simulink model "commqpskrx"  (R2013b)
settings: Solver=FixedStepDiscrete  SolverMode=SingleTasking  StartTime=0.0  StopTime=1-1e-05  RelTol=1e-3
PreLoadFcn:
  | qpsktxrx = commqpsktxrx_init1();
InitFcn:
  | FrameTime = qpsktxrx.Ts*qpsktxrx.FrameSize*qpsktxrx.Upsampling;
StopFcn:
  | if (strcmp(get_param('commqpskrx/Model Parameters','ShowRecvMsg'),'on'))
  |   if exist('received','var')
  |      commqpsktxrx_bits2char;
  |   else
  |      sprintf('%s\n%s\n%s\n%s','Please run the following two lines of code to get the message output:',...
  |       '>> received = <simOut>.get(''received'');',...
  |       '>> commqpsktxrx_bits2char;',...
  |       'where <simOut> is the output of the sim command.')
  |   end
  | end
undefined symbols (not defined in the file or in its folder): dfilt
libraries: simulink x4, dspsigops x4, commdigbbndpm3 x3, dspstat3 x3, dsparch4 x3, commrflib2 x2, commblksprivate x2, commsequence2 x2, commutil2 x2, commfilt2 x2, dspsrcs4 x2, commchan3 x1
(part 1 of 2)
CloseFcn:
  | clear interp_filter;
  | clear TED;
  | clear NCO_ctrl;
  | clear sdrqpsktxrx;
  | clear received;
  | clear qpsktxrx;
  | clear FrameTime;
Description:
  | QPSK Transmitter and Receiver.
  | 
  | This model shows the implementation of a QPSK transmitter and receiver.
settings Model: FPTRunName=Active  Creator=The MathWorks Inc.  LastModifiedBy=DPu1
settings DataIOCC: SignalLoggingSaveFormat=ModelDataLogs  SaveOutput=off  SaveTime=off
settings OptimizationCC: BooleanDataType=off  InlineParams=on  ExpressionDepthLimit=2147483647  LocalBlockOutputs=off
settings DebuggingCC: AlgebraicLoopMsg=error  MultiTaskDSMMsg=warning  MultiTaskCondExecSysMsg=none  SingleTaskRateTransMsg=error  ParameterPrecisionLossMsg=none  FcnCallInpInsideContextMsg=UseLocalSettings  StateNameClashWarn=warning
settings HardwareCC: TargetLongLongMode=on  TargetIntDivRoundTo=Zero  TargetEndianess=LittleEndian  TargetHWDeviceType=Generic->MATLAB Host Computer  ProdEqTarget=off
settings RTWCC: ProcessScript=grt_make_rtw_hook  IncludeERTFirstTime=on
settings GRTTargetCC: CodeReplacementLibrary=None  CombineOutputUpdateFcns=off  CPPClassGenCompliant=on

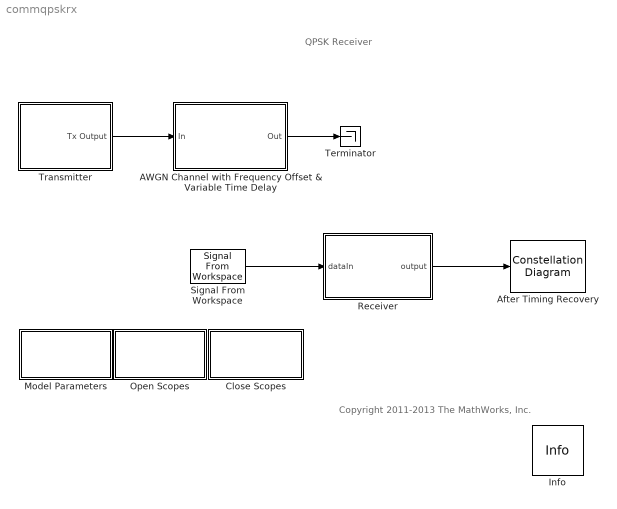
== system commqpskrx ==
  note: QPSK Receiver
  note: Copyright 2011-2013 The MathWorks, Inc.
  AWGN Channel with Frequency Offset & Variable Time Delay : Subsystem
      mask Display: disp('AWGN Channel with\nFrequency Offset & \nVariable Time Delay');
  After Timing Recovery : ConstellationDiagram  Tag=ScatterPlot
      settings: CopyFcn=scopeextensions.ScopeBlock.onCoreBlockCopy(gcbh);  DeleteFcn=scopeextensions.ScopeBlock.callback(gcbh, 'onBlockDelete');  PreSaveFcn=scopeextensions.ScopeBlock.callback(gcbh, 'onModelSave');  NameChangeFcn=scopeextensions.ScopeBlock.callback(gcbh, 'onBlockRename');  DestroyFcn=scopeextensions.ScopeBlock.onBlockDestroy(gcbh)  CloseFcn=scopeextensions.ScopeBlock.callback(gcbh, 'onBlockClose');  PreDeleteFcn=scopeextensions.ScopeBlock.callback(gcbh, 'onBlockPreDelete');
  Close Scopes : Subsystem
      settings: OpenFcn=|
      | % Close the Spectrum Scopes, Time Scopes, and the Scatter Plot Scopes
      | sdspfscope2([],[],[],'ScopeUpdate',[bdroot '/Transmitter/After RC Tx Filter'],'CloseFig');
      | set_param([bdroot '/Transmitter/After RC Tx Filter'],'OpenScopeAtSimStart','off');
      | 
      | channelSubsys = [bdroot '/AWGN Channel with Frequency Offset & Variable Time Delay'];
      | sdspfscope2([],[],[],'ScopeUpdate',[channelSubsys '/After Channel'],'CloseFig');
      | set_param([channelSubsys '/After Channel'],'OpenScopeAtSimStart','off');
      | 
      | TMW_Delay_TimeScope = scopeextensions.ScopeBlock.getInstance([channelSubsys '/Actual Delay']);
      | TMW_Delay_TimeScope.Visible = 'off';
      | TMW_Delay_TimeScope.ScopeCfg.OpenAtMdlStart = false;
      | 
      | sdspfscope2([],[],[],'ScopeUpdate',[bdroot '/Receiver/After RC Rx Filter'],'CloseFig');
      | set_param([bdroot '/Receiver/After RC Rx Filter'],'OpenScopeAtSimStart','off');
      | 
      | sdspfscope2([],[],[],'ScopeUpdate',[bdroot '/Receiver/After RC Rx Filter1'],'CloseFig');
      | set_param([bdroot '/Receiver/After RC Rx Filter1'],'OpenScopeAtSimStart','off');
      | 
      | CoarseFreqCompSubsys = [bdroot '/Receiver/Coarse Frequency Compensation'];
      | TMW_Freq_Offset_TimeScope = scopeextensions.ScopeBlock.getInstance([CoarseFreqCompSubsys '/Estimated Frequency Offset']);
      | TMW_Freq_Offset_TimeScope.Visible = 'off';
      | TMW_Freq_Offset_TimeScope.ScopeCfg.OpenAtMdlStart = false;
      | sdspfscope2([],[],[],'ScopeUpdate',[CoarseFreqCompSubsys '/Find Frequency Offset/After u^M'],'CloseFig');
      | set_param([CoarseFreqCompSubsys '/Find Frequency Offset/After u^M'],'OpenScopeAtSimStart','off');
      | % sdspfscope2([],[],[],'ScopeUpdate',[bdroot '/Receiver/After Coarse Frequency Compensation'],'CloseFig');
      | % set_param([bdroot '/Receiver/After Coarse Frequency Compensation'],'OpenScopeAtSimStart','off');
      | 
      | 
      | FineFreqCompSubsys = [bdroot '/Receiver/Fine Frequency Compensation'];
      | sdspfscope2([],[],[],'ScopeUpdate',[FineFreqCompSubsys '/Estimated Phase Difference'],'CloseFig');
      | set_param([FineFreqCompSubsys '/Estimated Phase Difference'],'OpenScopeAtSimStart','off');
      | 
      | sdspfscope2([],[],[],'ScopeUpdate',[bdroot '/Receiver/After Fine Frequency Compensation'],'CloseFig');
      | set_param([bdroot '/Receiver/After Fine Frequency Compensation'],'OpenScopeAtSimStart','off');
      | 
      | TimeRecSubsys = [bdroot '/Receiver/Timing Recovery'];
      | TMW_Delay_Offset_TimeScope = scopeextensions.ScopeBlock.getInstance([TimeRecSubsys '/Timing Recovery PLL/Normalized Timing Error']);
      | TMW_Delay_Offset_TimeScope.Visible = 'off';
      | TMW_Delay_Offset_TimeScope.ScopeCfg.OpenAtMdlStart = false;
      | 
      | sdspfscope2([],[],[],'ScopeUpdate',[TimeRecSubsys '/After Timing Recovery'],'CloseFig');
      | set_param([TimeRecSubsys '/After Timing Recovery'],'OpenScopeAtSimStart','off');
      | 
      | clear TMW_Delay_TimeScope TMW_Freq_Offset_TimeScope TMW_Delay_Offset_TimeScope;
      | clear channelSubsys CoarseFreqCompSubsys  FineFreqCompSubsys TimeRecSubsys;
      mask Display: disp('Double-click\nTo Close Scopes');
  Info : commblksprivate/Info  SystemSampleTime=-1
  Model Parameters : Subsystem  mask(Model Parameters){SettingCtrl=Timing recovery settings, EbN0dB=7, FreqOffset=5e3, DelayCtrl=Triangle, DelayStep=0.05, MinDelay=0, MaxDelay=8, DelayStart=0.1, FFTSize=2048, numSpecAverage=2, FineFreqNormalizedLoopBW=0.01, FineFreqDampingFactor=1, TimeRecNormalizedLoopBW=0.01, TimeRecDampingFactor=1, ShowRecvMsg=on}
      mask prompts: SettingCtrl "Setting types:"; EbN0dB "Eb/No (dB):"; FreqOffset "Frequency offset (Hz):"; DelayCtrl "Delay type:"; DelayStep "Delay step (samples/frame):"; MinDelay "Minimum delay (samples):"; MaxDelay "Maximum delay (samples):"; DelayStart "Start delay (samples):"; FFTSize "FFT size for coarse frequency compensation:"; numSpecAverage "Number of spectrum averages (frames):"; FineFreqNormalizedLoopBW "Normalized loop bandwidth:"; FineFreqDampingFactor "Damping factor:"; TimeRecNormalizedLoopBW "Normalized loop bandwidth:"; TimeRecDampingFactor "Damping factor:"; ShowRecvMsg "Show received message:"
      mask help: Choose to set the channel impairment parameters, FFT parameters for the coarse frequency compensation, PLL parameters for fine frequency compensation and timing recovery.
      mask init:
      | myException = commqpsktxrx_mask(gcb, 'init', DelayCtrl, MinDelay,...
      |     MaxDelay, DelayStart, DelayStep);
      | if ~isempty(myException)
      |    errordlg(myException.msg);
      | end
      mask Help: helpview(commdhelp);
      mask TypeOptions SettingCtrl: Channel impairment settings | FFT settings for coarse frequency compensation | Fine frequency compensation settings | Timing recovery settings
      mask Callback SettingCtrl: commqpsktxrx_mask(gcbh, 'cbShowHideSettingOptions');
      mask TypeOptions DelayCtrl: Ramp | Triangle
      mask Callback DelayCtrl: commqpsktxrx_mask(gcbh, 'cbShowHideDelayOptions');
      mask Display: disp('Model\nParameters');
  Open Scopes : Subsystem
      settings: OpenFcn=|
      | % Open the Spectrum Scopes, Time Scopes, and the Scatter Plot Scopes
      | sdspfscope2([],[],[],'ScopeUpdate',[bdroot '/Transmitter/After RC Tx Filter'],'OpenFig');
      | set_param([bdroot '/Transmitter/After RC Tx Filter'],'OpenScopeAtSimStart','on');
      | 
      | sdspfscope2([],[],[],'ScopeUpdate',[bdroot '/AWGN Channel with Frequency Offset & Variable Time Delay/After Channel'],'OpenFig');
      | set_param([bdroot '/AWGN Channel with Frequency Offset & Variable Time Delay/After Channel'],'OpenScopeAtSimStart','on');
      | 
      | channelSubsys = [bdroot '/AWGN Channel with Frequency Offset & Variable Time Delay'];
      | TMW_Delay_TimeScope = scopeextensions.ScopeBlock.getInstance([channelSubsys '/Actual Delay']);
      | TMW_Delay_TimeScope.Visible = 'on';
      | TMW_Delay_TimeScope_hs = TMW_Delay_TimeScope.Framework;
      | % Enable the Plot Navigation
      | TMW_Delay_TimeScope_hs.ExtDriver.ConfigDb.findConfig('Tools', 'Plot Navigation').Enable = true;
      | TMW_Delay_TimeScope.Position = figposition([1.5 6.3 22 24]);
      | TMW_Delay_TimeScope.ScopeCfg.OpenAtMdlStart = true;
      | 
      | sdspfscope2([],[],[],'ScopeUpdate',[bdroot '/Receiver/After RC Rx Filter'],'OpenFig');
      | set_param([bdroot '/Receiver/After RC Rx Filter'],'OpenScopeAtSimStart','on');
      | 
      | sdspfscope2([],[],[],'ScopeUpdate',[bdroot '/Receiver/After RC Rx Filter1'],'OpenFig');
      | set_param([bdroot '/Receiver/After RC Rx Filter1'],'OpenScopeAtSimStart','on');
      | 
      | CoarseFreqCompSubsys = [bdroot '/Receiver/Coarse Frequency Compensation'];
      | TMW_Freq_Offset_TimeScope = scopeextensions.ScopeBlock.getInstance([CoarseFreqCompSubsys '/Estimated Frequency Offset']);
      | TMW_Freq_Offset_TimeScope.Visible = 'on';
      | TMW_Freq_Offset_TimeScope_hs = TMW_Freq_Offset_TimeScope.Framework;
      | % Enable the Plot Navigation
      | TMW_Freq_Offset_TimeScope_hs.ExtDriver.ConfigDb.findConfig('Tools', 'Plot Navigation').Enable = true;
      | TMW_Freq_Offset_TimeScope.Position = figposition([24 6.3 22 24]);
      | TMW_Freq_Offset_TimeScope.ScopeCfg.OpenAtMdlStart = true;
      | sdspfscope2([],[],[],'ScopeUpdate',[CoarseFreqCompSubsys '/Find Frequency Offset/After u^M'],'OpenFig');
      | set_param([CoarseFreqCompSubsys '/Find Frequency Offset/After u^M'],'OpenScopeAtSimStart','on');
      | % sdspfscope2([],[],[],'ScopeUpdate',[bdroot '/Receiver/After Coarse Frequency Compensation'],'OpenFig');
      | % set_param([bdroot '/Receiver/After Coarse Frequency Compensation'],'OpenScopeAtSimStart','on');
      | 
      | 
      | FineFreqCompSubsys = [bdroot '/Receiver/Fine Frequency Compensation'];
      | sdspfscope2([],[],[],'ScopeUpdate',[FineFreqCompSubsys '/Estimated Phase Difference'],'OpenFig');
      | set_param([FineFreqCompSubsys '/Estimated Phase Difference'],'OpenScopeAtSimStart','on');
      | 
      | sdspfscope2([],[],[],'ScopeUpdate',[bdroot '/Receiver/After Fine Frequency Compensation'],'OpenFig');
      | set_param([bdroot '/Receiver/After Fine Frequency Compensation'],'OpenScopeAtSimStart','on');
      | 
      | TimeRecSubsys = [bdroot '/Receiver/Timing Recovery'];
      | TMW_Delay_Offset_TimeScope = scopeextensions.ScopeBlock.getInstance([TimeRecSubsys '/Timing Recovery PLL/Normalized Timing Error']);
      | TMW_Delay_Offset_TimeScope.Visible = 'on';
      | TMW_Delay_Offset_TimeScope_hs = TMW_Delay_Offset_TimeScope.Framework;
      | % Enable the Plot Navigation
      | TMW_Delay_Offset_TimeScope_hs.ExtDriver.ConfigDb.findConfig('Tools', 'Plot Navigation').Enable = true;
      | TMW_Delay_Offset_TimeScope.Position = figposition([46.5 6.3 22 24]);
      | TMW_Delay_Offset_TimeScope.ScopeCfg.OpenAtMdlStart = true;
      | 
      | sdspfscope2([],[],[],'ScopeUpdate',[TimeRecSubsys '/After Timing Recovery'],'OpenFig');
      | set_param([TimeRecSubsys '/After Timing Recovery'],'OpenScopeAtSimStart','on');
      | clear TMW_Delay_TimeScope TMW_Freq_Offset_TimeScope TMW_Delay_Offset_TimeScope TMW_Delay_TimeScope_hs TMW_Freq_Offset_TimeScope_hs TMW_Delay_Offset_TimeScope_hs;
      | clear channelSubsys CoarseFreqCompSubsys  FineFreqCompSubsys TimeRecSubsys;
      mask Display: disp('Double-click\nTo Open Scopes\nAt Run Time');
  Receiver : Subsystem
      mask Display: disp('Receiver')
  Signal From Workspace : dspsrcs4/Signal From Workspace  X=rxsignal  Ts=0.002/400  nsamps=400  OutputAfterFinalValue=Cyclic repetition  ignoreOrWarnInputAndFrameLengths=off
  Terminator : Terminator
  Transmitter : Subsystem
      mask Display: disp('Transmitter')
  wires:
  Transmitter/1(Tx Output) -> AWGN Channel with Frequency Offset & Variable Time Delay/1(In)
  AWGN Channel with Frequency Offset & Variable Time Delay/1(Out) -> Terminator/1
  Signal From Workspace/1 -> Receiver/1(dataIn)
  Receiver/1(output) -> After Timing Recovery/1

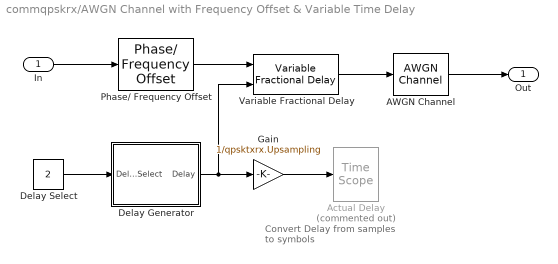
== system commqpskrx/AWGN Channel with Frequency Offset & Variable Time Delay ==
  note: Convert Delay from
      | samples to symbols
  In : Inport
  AWGN Channel : commchan3/AWGN Channel  InputProcessing=Inherited (this choice will be removed - see release notes)  seed=67  noiseMode="Signal to noise ratio  (Eb/No)"  EbNodB=7  EsNodB=15  SNRdB=15  bitsPerSym=2  Ps=1/qpsktxrx.Upsampling  Tsym=qpsktxrx.Upsampling*qpsktxrx.Ts  variance=1
  Actual Delay : TimeScope  Commented=on  DefaultConfigurationName=spbscopes.TimeScopeBlockCfg
      settings: CopyFcn=scopeextensions.ScopeBlock.onCoreBlockCopy(gcbh);  DeleteFcn=scopeextensions.ScopeBlock.callback(gcbh, 'onBlockDelete');  PreSaveFcn=scopeextensions.ScopeBlock.callback(gcbh, 'onModelSave');  NameChangeFcn=scopeextensions.ScopeBlock.callback(gcbh, 'onBlockRename');  DestroyFcn=scopeextensions.ScopeBlock.onBlockDestroy(gcbh)  CloseFcn=scopeextensions.ScopeBlock.callback(gcbh, 'onBlockClose');  PreDeleteFcn=scopeextensions.ScopeBlock.callback(gcbh, 'onBlockPreDelete');
  Delay Generator : Subsystem
      mask Display: disp('Delay Generator')
  Delay Select : Constant  Value=2
  Gain : Gain  Gain=1/qpsktxrx.Upsampling
  Phase/ Frequency Offset : commrflib2/Phase// Frequency Offset  phaseOffset=qpsktxrx.PhaseOffset  freqPort=off  freqOffset=5000
  Variable Fractional Delay : dspsigops/Variable Fractional Delay  mode=OBSOLETE  modeActive=Linear  dmax=qpsktxrx.FrameSize*qpsktxrx.Upsampling  InputProcessing=Columns as channels (frame based)  L=4  FarrowL=4  R=10  alpha=1  ic=0  fallbackFIR=Clip to the minimum value necessary for centered kernel  fallbackFarrow=Clip to the minimum value necessary for centered kernel  noDFT=off  roundingMode=Zero  overflowMode=off
  Out : Outport
  wires:
  AWGN Channel/1 -> Out/1
  In/1 -> Phase/ Frequency Offset/1
  Phase/ Frequency Offset/1 -> Variable Fractional Delay/1
  Variable Fractional Delay/1 -> AWGN Channel/1
  Delay Select/1 -> Delay Generator/1(Delay Select)
  Delay Generator/1(Delay) -> Variable Fractional Delay/2, Gain/1
  Gain/1 -> Actual Delay/1

== system commqpskrx/Close Scopes ==

== system commqpskrx/Model Parameters ==

== system commqpskrx/Open Scopes ==

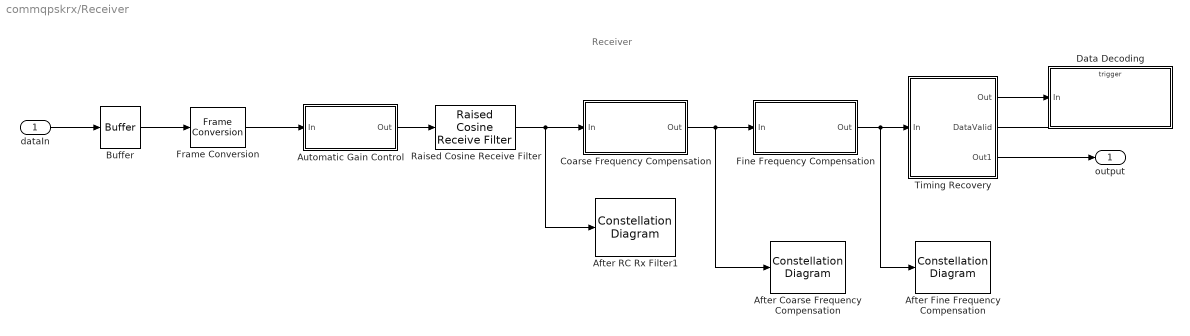
== system commqpskrx/Receiver ==
  note: Receiver
  dataIn : Inport
  After Coarse Frequency Compensation : ConstellationDiagram  Tag=ScatterPlot
      settings: CopyFcn=scopeextensions.ScopeBlock.onCoreBlockCopy(gcbh);  DeleteFcn=scopeextensions.ScopeBlock.callback(gcbh, 'onBlockDelete');  PreSaveFcn=scopeextensions.ScopeBlock.callback(gcbh, 'onModelSave');  NameChangeFcn=scopeextensions.ScopeBlock.callback(gcbh, 'onBlockRename');  DestroyFcn=scopeextensions.ScopeBlock.onBlockDestroy(gcbh)  CloseFcn=scopeextensions.ScopeBlock.callback(gcbh, 'onBlockClose');  PreDeleteFcn=scopeextensions.ScopeBlock.callback(gcbh, 'onBlockPreDelete');
  After Fine Frequency Compensation : ConstellationDiagram  Tag=ScatterPlot
      settings: CopyFcn=scopeextensions.ScopeBlock.onCoreBlockCopy(gcbh);  DeleteFcn=scopeextensions.ScopeBlock.callback(gcbh, 'onBlockDelete');  PreSaveFcn=scopeextensions.ScopeBlock.callback(gcbh, 'onModelSave');  NameChangeFcn=scopeextensions.ScopeBlock.callback(gcbh, 'onBlockRename');  DestroyFcn=scopeextensions.ScopeBlock.onBlockDestroy(gcbh)  CloseFcn=scopeextensions.ScopeBlock.callback(gcbh, 'onBlockClose');  PreDeleteFcn=scopeextensions.ScopeBlock.callback(gcbh, 'onBlockPreDelete');
  After RC Rx Filter1 : ConstellationDiagram  Tag=ScatterPlot
      settings: CopyFcn=scopeextensions.ScopeBlock.onCoreBlockCopy(gcbh);  DeleteFcn=scopeextensions.ScopeBlock.callback(gcbh, 'onBlockDelete');  PreSaveFcn=scopeextensions.ScopeBlock.callback(gcbh, 'onModelSave');  NameChangeFcn=scopeextensions.ScopeBlock.callback(gcbh, 'onBlockRename');  DestroyFcn=scopeextensions.ScopeBlock.onBlockDestroy(gcbh)  CloseFcn=scopeextensions.ScopeBlock.callback(gcbh, 'onBlockClose');  PreDeleteFcn=scopeextensions.ScopeBlock.callback(gcbh, 'onBlockPreDelete');
  Automatic Gain Control : Subsystem  mask{DesiredAmplitude=1/sqrt(qpsktxrx.Upsampling)}
      mask prompts: DesiredAmplitude "Desired Amplitude"
      mask Display: disp('Automatic Gain\nControl')
  Buffer : Buffer  N=qpsktxrx.RxBufferedFrames*qpsktxrx.FrameSize*qpsktxrx.Upsampling  TreatMby1Signals=One channel
  Coarse Frequency Compensation : Subsystem
      mask Display: disp('Coarse Frequency\nCompensation');
  Data Decoding : Subsystem
      mask Display: disp('Data Decoding');
  Fine Frequency Compensation : Subsystem
      mask Display: disp('Fine Frequency\nCompensation')
  Frame Conversion : FrameConversion  OutFrame=Sample-based
  Raised Cosine Receive Filter : commfilt2/Raised Cosine Receive Filter  filtType=Square root  N=qpsktxrx.Upsampling  filtSpan=qpsktxrx.RaisedCosineFilterSpan  currentFiltSpan=qpsktxrx.RaisedCosineFilterSpan  D=(qpsktxrx.RaisedCosineFilterSpan)/2  R=0.5  sampMode=Mute  saveAsFlag=0  rateMode=Downsampling  downFactor=qpsktxrx.Downsampling  downOffset=0  framing=Enforce single-rate processing  InputProcessing=Columns as channels (frame based)  checkGain=Normalized  filterGain=1  checkCoeff=off  variableName=rcRxFilt1  launchFVT=off  roundingMode=Floor  overflowMode=off
  Timing Recovery : Subsystem
      mask Display:
      | disp('Timing\nRecovery');
      | port_label('output',1,'DataOut');
      | port_label('output',2,'DataValid');
  output : Outport
  wires:
  Timing Recovery/1(Out) -> Data Decoding/1(In)
  dataIn/1 -> Buffer/1
  Timing Recovery/2(DataValid) -> Data Decoding/Trigger
  Raised Cosine Receive Filter/1 -> Coarse Frequency Compensation/1(In), After RC Rx Filter1/1
  Coarse Frequency Compensation/1(Out) -> Fine Frequency Compensation/1(In), After Coarse Frequency Compensation/1
  Fine Frequency Compensation/1(Out) -> Timing Recovery/1(In), After Fine Frequency Compensation/1
  Buffer/1 -> Frame Conversion/1
  Frame Conversion/1 -> Automatic Gain Control/1(In)
  Automatic Gain Control/1(Out) -> Raised Cosine Receive Filter/1
  Timing Recovery/3(Out1) -> output/1

== system commqpskrx/Transmitter ==
  note: Transmitter
  Bit Generation : Subsystem
      mask Display: disp('Bits Generation')
  QPSK Modulator Baseband : commdigbbndpm3/QPSK Modulator Baseband  InType=Bit  Enc=Gray  Ph=pi/4  outDtype=double  outWordLen=16  outUDDataType=sfix(16)  outFracLenMode=Best precision  outFracLen=15
  Raised Cosine Transmit Filter : commfilt2/Raised Cosine Transmit Filter  filtType=Square root  filtSpan=qpsktxrx.RaisedCosineFilterSpan  currentFiltSpan=qpsktxrx.RaisedCosineFilterSpan  D=(qpsktxrx.RaisedCosineFilterSpan)/2  R=0.5  sampMode=Mute  saveAsFlag=0  N=qpsktxrx.Upsampling  framing=Enforce single-rate processing  InputProcessing=Columns as channels (frame based)  checkGain=Normalized  filterGain=1  checkCoeff=off  variableName=rcTxFilt  launchFVT=off  roundingMode=Floor  overflowMode=off
  Tx Output : Outport
  wires:
  Bit Generation/1(Out) -> QPSK Modulator Baseband/1
  QPSK Modulator Baseband/1 -> Raised Cosine Transmit Filter/1
  Raised Cosine Transmit Filter/1 -> Tx Output/1

== system commqpskrx/AWGN Channel with Frequency Offset & Variable Time Delay/Delay Generator ==
  Delay Select : Inport
  Multiport Switch : MultiPortSwitch  Inputs=2  OutDataTypeStr=double
  Repeating Sequence Stair : simulink/Sources/Repeating Sequence Stair  OutValues="[0        0.05         0.1        0.15         0.2        0.25         0.3        0.35         0.4        0.45         0.5        0.55         0.6        0.65         0.7        0.75         0.8        0.85         0.9        0.95           1        1.05         1.1        1.15         1.2        1.25         1.3        1.35         1.4        1.45         1.5        1.55         1.6        1.65         1.7        1.75         1.8        1.85         1.9        1.95           2        2.05         2.1        2.15         2.2        2.25         2.3        2.35         2.4        2.45         2.5        2.55         2.6        2.65         2.7        2.75         2.8        2.85         2.9        2.95           3        3.05         3.1        3.15         3.2        3.25         3.3        3.35         3.4        3.45         3.5        3.55         3.6        3.65         3.7        3.75         3.8        3.85         3.9        3.95           4        4.05         4.1        4.15         4.2        4.25         4.3        4.35         4.4        4.45         4.5        4.55         4.6        4.65         4.7        4.75         4.8        4.85         4.9        4.95           5        5.05         5.1        5.15         5.2        5.25         5.3        5.35         5.4        5.45         5.5        5.55         5.6        5.65         5.7        5.75         5.8        5.85         5.9        5.95           6        6.05         6.1        6.15         6.2        6.25         6.3        6.35         6.4        6.45         6.5        6.55         6.6        6.65         6.7        6.75         6.8        6.85         6.9        6.95           7        7.05         7.1        7.15         7.2        7.25         7.3        7.35         7.4        7.45         7.5        7.55         7.6        7.65         7.7        7.75         7.8        7.85         7.9        7.95           8        7.95         7.9        7.85         7.8        7.75         7.7        7.65         7.6        7.55         7.5        7.45         7.4        7.35         7.3        7.25         7.2        7.15         7.1        7.05           7        6.95         6.9        6.85         6.8        6.75         6.7        6.65         6.6        6.55         6.5        6.45         6.4        6.35         6.3        6.25         6.2        6.15         6.1        6.05           6        5.95         5.9        5.85         5.8        5.75         5.7        5.65         5.6        5.55         5.5        5.45         5.4        5.35         5.3        5.25         5.2        5.15         5.1        5.05           5        4.95         4.9        4.85         4.8        4.75         4.7        4.65         4.6        4.55         4.5        4.45         4.4        4.35         4.3        4.25         4.2        4.15         4.1        4.05           4        3.95         3.9        3.85         3.8        3.75         3.7        3.65         3.6        3.55         3.5        3.45         3.4        3.35         3.3        3.25         3.2        3.15         3.1        3.05           3        2.95         2.9        2.85         2.8        2.75         2.7        2.65         2.6        2.55         2.5        2.45         2.4        2.35         2.3        2.25         2.2        2.15         2.1        2.05           2        1.95         1.9        1.85         1.8        1.75         1.7        1.65         1.6        1.55         1.5        1.45         1.4        1.35         1.3        1.25         1.2        1.15         1.1        1.05           1        0.95         0.9        0.85         0.8        0.75         0.7        0.65         0.6        0.55         0.5        0.45         0.4        0.35         0.3        0.25         0.2        0.15         0.1        0.05]"  tsamp=qpsktxrx.FrameSize*qpsktxrx.Upsampling*qpsktxrx.Ts  OutMin=[]  OutMax=[]  OutDataTypeStr=double  OutputDataTypeScalingMode=double  OutDataType=fixdt(0,8)  ConRadixGroup=Best Precision: Vector-wise  OutScaling=2^-12
  mVariableRamp : Subsystem
  Delay : Outport
  wires:
  Delay Select/1 -> Multiport Switch/1
  Repeating Sequence Stair/1 -> Multiport Switch/3
  mVariableRamp/1(Out) -> Multiport Switch/2
  Multiport Switch/1 -> Delay/1

== system commqpskrx/Receiver/Automatic Gain Control ==
  In : Inport
  AGC : commrfcorlib/AGC  SimulateUsing=Interpreted execution  DetectorMethod=Rectifier  LoopMethod=Linear  UpdatePeriod=32  StepSize=0.5  MaximumGain=20  GainOutputPort=off
  Gain : Gain  Gain=DesiredAmplitude
  Out : Outport
  wires:
  In/1 -> AGC/1
  Gain/1 -> Out/1
  AGC/1 -> Gain/1

== system commqpskrx/Receiver/Coarse Frequency Compensation ==
  In : Inport
  Compensate for Frequency Offset : commrflib2/Phase// Frequency Offset  phaseOffset=0  freqPort=on  freqOffset=100
  Estimated Frequency Offset : TimeScope  Commented=on  DefaultConfigurationName=spbscopes.TimeScopeBlockCfg
      settings: CopyFcn=scopeextensions.ScopeBlock.onCoreBlockCopy(gcbh);  DeleteFcn=scopeextensions.ScopeBlock.callback(gcbh, 'onBlockDelete');  PreSaveFcn=scopeextensions.ScopeBlock.callback(gcbh, 'onModelSave');  NameChangeFcn=scopeextensions.ScopeBlock.callback(gcbh, 'onBlockRename');  DestroyFcn=scopeextensions.ScopeBlock.onBlockDestroy(gcbh)  CloseFcn=scopeextensions.ScopeBlock.callback(gcbh, 'onBlockClose');  PreDeleteFcn=scopeextensions.ScopeBlock.callback(gcbh, 'onBlockPreDelete');
  Find Frequency Offset : Subsystem
  Gain : Gain  Gain=-1
  Out : Outport
  wires:
  Find Frequency Offset/1(Freq Offset) -> Gain/1, Estimated Frequency Offset/1
  In/1 -> Compensate for Frequency Offset/1, Find Frequency Offset/1(In)
  Compensate for Frequency Offset/1 -> Out/1
  Gain/1 -> Compensate for Frequency Offset/2

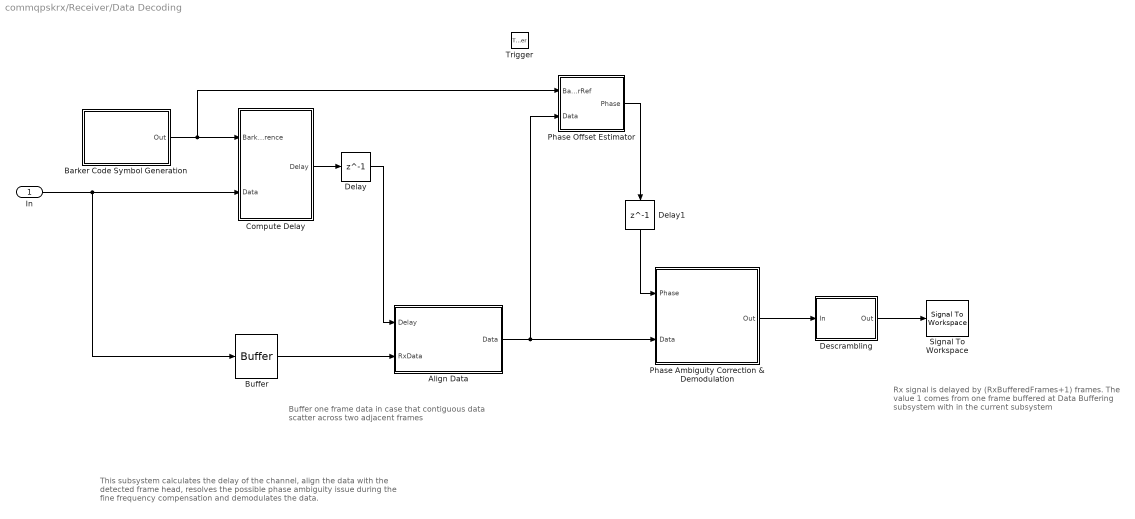
== system commqpskrx/Receiver/Data Decoding ==
  note: Buffer one frame data in case that contiguous
      | data scatter across two adjacent frames
  note: This subsystem calculates the delay of the channel, align the data with
      | the detected frame head, resolves the possible phase ambiguity issue
      | during the fine frequency compensation and demodulates the data.
  note: Rx signal is delayed by (RxBufferedFrames+1) frames.
      | The value 1 comes from one frame buffered at Data
      | Buffering subsystem with in the current subsystem
  In : Inport
  Trigger : TriggerPort  PortDimensions=1
  Align Data : MATLAB Function  TreatAsAtomicUnit=on
  "Barker Code Symbol Generation " : Subsystem
      mask Display: disp('Barker Code\nSymbol Generation')
  Buffer : Buffer  N=qpsktxrx.FrameSize*2  V=qpsktxrx.FrameSize  TreatMby1Signals=One channel
  Compute Delay : Subsystem
      mask Display: disp('Compute\nDelay');
  Delay : Delay  DelayLength=1
  Delay1 : Delay  DelayLength=1
  Descrambling : Subsystem
      mask Display: disp('Descrambling');
  Phase Ambiguity Correction & Demodulation : Subsystem
      mask Display: disp('Phase Ambiguity\nCorrection\n& Demodulation');
  Phase Offset Estimator : Subsystem
  Signal To Workspace : SignalToWorkspace  VariableName=received
      settings: CopyFcn=dspblkcopystw(gcbh);
  wires:
  Delay/1 -> Align Data/1(Delay)
  Buffer/1 -> Align Data/2(RxData)
  In/1 -> Compute Delay/2(Data), Buffer/1
  Compute Delay/1(Delay) -> Delay/1
  Align Data/1(Data) -> Phase Ambiguity Correction & Demodulation/2(Data), Phase Offset Estimator/2(Data)
  Phase Ambiguity Correction & Demodulation/1(Out) -> Descrambling/1(In)
  "Barker Code Symbol Generation "/1(Out) -> Compute Delay/1(Barker Reference), Phase Offset Estimator/1(BarkerRef)
  Phase Offset Estimator/1(Phase) -> Delay1/1
  Delay1/1 -> Phase Ambiguity Correction & Demodulation/1(Phase)
  Descrambling/1(Out) -> Signal To Workspace/1

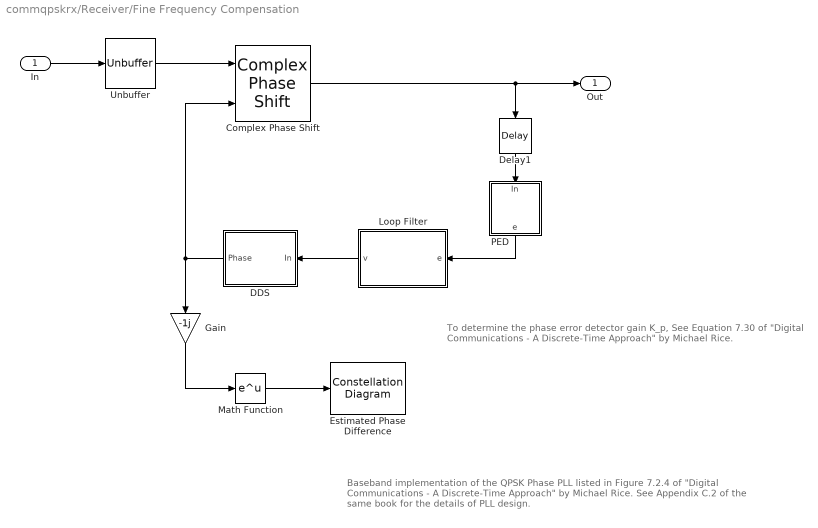
== system commqpskrx/Receiver/Fine Frequency Compensation ==
  note: To determine the phase error detector gain K_p, See Equation 7.30 of "Digital
      | Communications - A Discrete-Time Approach" by Michael Rice.
  note: Baseband implementation of the QPSK Phase PLL listed in Figure 7.2.4 of
      | "Digital Communications - A Discrete-Time Approach" by Michael Rice. See
      | Appendix C.2 of the same book for the details of PLL design.
  In : Inport
  Complex Phase Shift : commutil2/Complex Phase Shift
  DDS : Subsystem
      mask Display: disp('DDS')
  Delay1 : dspsigops/Delay  InputProcessing=Columns as channels (frame based)  dly_unit=Samples  delay=1  ic_detail=off  dif_ic_for_ch=off  dif_ic_for_dly=off  ic=0  reset_popup=None
  Estimated Phase Difference : ConstellationDiagram  Tag=ScatterPlot
      settings: CopyFcn=scopeextensions.ScopeBlock.onCoreBlockCopy(gcbh);  DeleteFcn=scopeextensions.ScopeBlock.callback(gcbh, 'onBlockDelete');  PreSaveFcn=scopeextensions.ScopeBlock.callback(gcbh, 'onModelSave');  NameChangeFcn=scopeextensions.ScopeBlock.callback(gcbh, 'onBlockRename');  DestroyFcn=scopeextensions.ScopeBlock.onBlockDestroy(gcbh)  CloseFcn=scopeextensions.ScopeBlock.callback(gcbh, 'onBlockClose');  PreDeleteFcn=scopeextensions.ScopeBlock.callback(gcbh, 'onBlockPreDelete');
  Gain : Gain  Gain=-1j
  Loop Filter : Subsystem  mask{BnTs=0.01, zeta=1, N=qpsktxrx.Upsampling/qpsktxrx.Downsampling, Kp=qpsktxrx.PhaseErrorDetectorGain, K0=qpsktxrx.PhaseRecoveryGain}
      mask prompts: BnTs "Normalized Loop Bandwidth"; zeta "Damping Factor"; N "Number of Samples/Symbol"; Kp "Phase Detector Gain (Kp)"; K0 "DDS Gain (K0)"
      mask init:
      | % See C.57 to C.61 in Michael Rice's "Digital Communications 
      | % - A Discrete-Time Approach" for details
      | theta = BnTs/(zeta+0.25/zeta)/N;
      | d = 1 + 2*zeta*theta + theta*theta;
      | K1 = 4*zeta*theta/d;
      | K2 = 4*theta*theta/d;
      | K1 = K1/(Kp*K0);
      | K2 = K2/(Kp*K0);
      mask Display: disp('Loop Filter')
  Math Function : Math  SaturateOnIntegerOverflow=on
  PED : MATLAB Function  TreatAsAtomicUnit=on
  Unbuffer : Unbuffer  SampleBasedProcessing=Same as frame based
  Out : Outport
  wires:
  Gain/1 -> Math Function/1
  Math Function/1 -> Estimated Phase Difference/1
  PED/1(e) -> Loop Filter/1(e)
  Loop Filter/1(v) -> DDS/1(In)
  DDS/1(Phase) -> Complex Phase Shift/2, Gain/1
  In/1 -> Unbuffer/1
  Complex Phase Shift/1 -> Delay1/1, Out/1
  Delay1/1 -> PED/1(In)
  Unbuffer/1 -> Complex Phase Shift/1

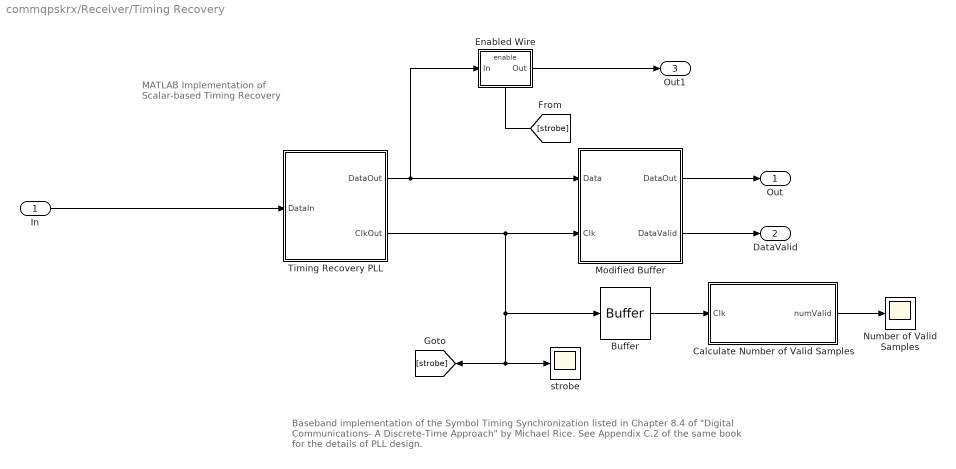
== system commqpskrx/Receiver/Timing Recovery ==
  note: Baseband implementation of the Symbol Timing Synchronization listed in Chapter 8.4
      | of "Digital Communications- A Discrete-Time Approach" by Michael Rice. See
      | Appendix C.2 of the same book for the details of PLL design.
  note: MATLAB Implementation
      | of Scalar-based Timing Recovery
  In : Inport
  Buffer : Buffer  N=qpsktxrx.FrameSize*qpsktxrx.Upsampling/qpsktxrx.Downsampling  TreatMby1Signals=One channel
  Calculate Number of Valid Samples : MATLAB Function  TreatAsAtomicUnit=on
  Enabled Wire : Subsystem  TreatAsAtomicUnit=on
  Modified Buffer : Subsystem  TreatAsAtomicUnit=on  mask(Input-Driven Buffer){bufSize=qpsktxrx.FrameSize}
      mask prompts: bufSize "Buffer size:"
      mask help: A modified buffer subsystem that is driven by the arrival of its input data; it produces a valid output data buffer whenever its buffer is full and sets its dataValid flag to 1. Otherwise, the data at its dataOut port is not valid and its dataValid flag is set to 0.
      mask Display: disp('Modified Buffer')
  Number of Valid Samples : Scope
      settings: TimeRange=0.1  YMin=95  YMax=105  SaveName=ScopeData3  MaxDataPoints=50000
  Timing Recovery PLL : Subsystem
      mask Display:
      | disp('Timing Recovery\nPLL')
      | port_label('input',1,'In')
      | port_label('output',1,'DataOut')
      | port_label('output',2,'Clk')
  strobe : Scope
  Out : Outport
  DataValid : Outport  Port=2
  Out1 : Outport  Port=3
  wires:
  Timing Recovery PLL/2(ClkOut) -> [strobe], strobe/1, Buffer/1, Modified Buffer/2(Clk)
  Timing Recovery PLL/1(DataOut) -> Enabled Wire/1(In), Modified Buffer/1(Data)
  Calculate Number of Valid Samples/1(numValid) -> Number of Valid Samples/1
  [strobe] -> Enabled Wire/Enable
  In/1 -> Timing Recovery PLL/1(DataIn)
  Modified Buffer/1(DataOut) -> Out/1
  Modified Buffer/2(DataValid) -> DataValid/1
  Buffer/1 -> Calculate Number of Valid Samples/1(Clk)
  Enabled Wire/1(Out) -> Out1/1

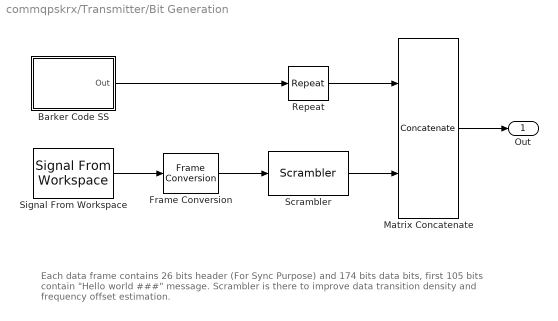
== system commqpskrx/Transmitter/Bit Generation ==
  note: Each data frame contains 26 bits header (For Sync Purpose) and 174 bits data bits,
      | first 105 bits contain "Hello world ###" message. Scrambler is there to improve data
      | transition density and frequency offset estimation.
  Barker Code SS : Subsystem
      mask Display: disp('Unipolar\nBarker Code')
  Frame Conversion : FrameConversion  OutFrame=Sample-based
  Matrix Concatenate : Concatenate  Mode=Multidimensional array
  Repeat : dspsigops/Repeat  N=2  InputProcessing=Columns as channels (frame based)  RateOptions=Enforce single-rate processing  ic=0  mode=Unused parameter value
  Scrambler : commsequence2/Scrambler  M=2  poly=[1 1 1 0 1]  ini_sta=[0 0 0 0]
  Signal From Workspace : dspsrcs4/Signal From Workspace  X=qpsktxrx.sBit  Ts=1/qpsktxrx.DataLength*FrameTime  nsamps=qpsktxrx.DataLength  OutputAfterFinalValue=Cyclic repetition  ignoreOrWarnInputAndFrameLengths=off
  Out : Outport
  wires:
  Barker Code SS/1(Out) -> Repeat/1
  Matrix Concatenate/1 -> Out/1
  Signal From Workspace/1 -> Frame Conversion/1
  Repeat/1 -> Matrix Concatenate/1
  Scrambler/1 -> Matrix Concatenate/2
  Frame Conversion/1 -> Scrambler/1

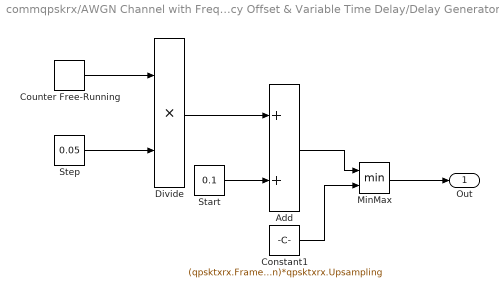
== system commqpskrx/AWGN Channel with Frequency Offset & Variable Time Delay/Delay Generator/mVariableRamp ==
  Add : Sum
  Constant1 : Constant  Value=(qpsktxrx.FrameSize-qpsktxrx.RaisedCosineFilterSpan)*qpsktxrx.Upsampling
  Counter Free-Running : simulink/Sources/Counter Free-Running  NumBits=64  tsamp=qpsktxrx.FrameSize*qpsktxrx.Upsampling*qpsktxrx.Ts
  Divide : Product  Inputs=**
  MinMax : MinMax  Inputs=2
  Start : Constant  Value=0.1
  Step : Constant  Value=0.05
  Out : Outport
  wires:
  Counter Free-Running/1 -> Divide/1
  Step/1 -> Divide/2
  Divide/1 -> Add/1
  Start/1 -> Add/2
  Add/1 -> MinMax/1
  MinMax/1 -> Out/1
  Constant1/1 -> MinMax/2

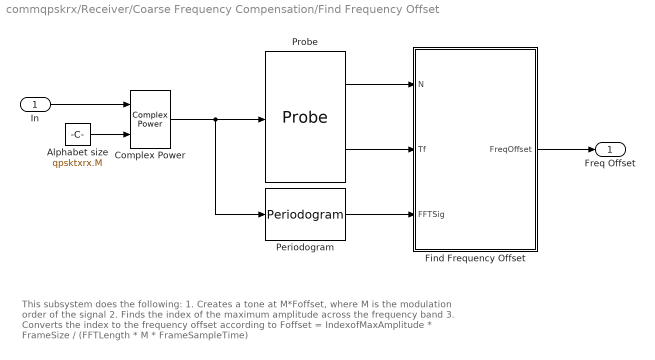
== system commqpskrx/Receiver/Coarse Frequency Compensation/Find Frequency Offset ==
  note: This subsystem does the following:
      | 1.  Creates a tone at M*Foffset, where M is the modulation order of the signal
      | 2.  Finds the index of the maximum amplitude across the frequency band
      | 3.  Converts the index to the frequency offset according to
      | Foffset = IndexofMaxAmplitude * FrameSize / (FFTLength * M * FrameSampleTime)
  In : Inport
  Alphabet size : Constant  Value=qpsktxrx.M  OutDataTypeStr=Inherit: Inherit via back propagation
  Complex Power : commblksprivate/Complex Power
  Find Frequency Offset : MATLAB Function  TreatAsAtomicUnit=on
  Periodogram : dspspect3/Periodogram  measurement=Power spectral density  wintype=Hamming  Rs=50  beta=5  winsamp=Symmetric  FFTImplementation=Auto  inheritFFT=off  fftsize=2048  navg=2  inheritTs=on  Ts=1
  Probe : Probe  ProbeComplexSignal=off
  Freq Offset : Outport
  wires:
  Periodogram/1 -> Find Frequency Offset/3(FFTSig)
  Alphabet size/1 -> Complex Power/2
  In/1 -> Complex Power/1
  Probe/1 -> Find Frequency Offset/1(N)
  Probe/2 -> Find Frequency Offset/2(Tf)
  Find Frequency Offset/1(FreqOffset) -> Freq Offset/1
  Complex Power/1 -> Probe/1, Periodogram/1

== system commqpskrx/Receiver/Data Decoding/Barker Code Symbol Generation  ==
  note: Regenerate a QPSK-modulated unipolar Barker code sequence
      | to be compared with the received data
  Constant Barker Code : Constant  Value=|  VectorParams1D=off  OutDataTypeStr=double
      | [+1 +1 +1 +1 +1 -1 -1 +1 +1 -1 +1 -1 +1
      | ].' > 0
  QPSK Modulator Baseband : commdigbbndpm3/QPSK Modulator Baseband  InType=Bit  Enc=Gray  Ph=pi/4  outDtype=double  outWordLen=16  outUDDataType=sfix(16)  outFracLenMode=Best precision  outFracLen=15
  Repeat : dspsigops/Repeat  N=2  InputProcessing=Columns as channels (frame based)  RateOptions=Enforce single-rate processing  ic=0  mode=Unused parameter value
  Out : Outport
  wires:
  Constant Barker Code/1 -> Repeat/1
  Repeat/1 -> QPSK Modulator Baseband/1
  QPSK Modulator Baseband/1 -> Out/1

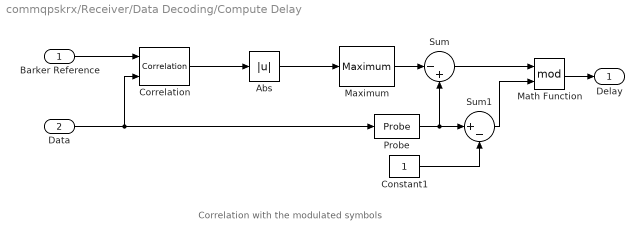
== system commqpskrx/Receiver/Data Decoding/Compute Delay ==
  note: Correlation with the modulated symbols
  Barker Reference : Inport
  Data : Inport  Port=2
  Abs : Abs
  Constant1 : Constant  VectorParams1D=off  OutDataTypeStr=Inherit: Inherit via back propagation  FramePeriod=2
  Correlation : dspstat3/Correlation  domain=Time  outputDataTypeStr=Inherit: Same as accumulator  outputLastDataTypeStr=Inherit: Same as accumulator  outputMin=[]  outputMax=[]  accumDataTypeStr=Inherit: Same as product output  accumLastDataTypeStr=Inherit: Same as product output  roundingMode=Floor  overflowMode=off
  Math Function : Math  Operator=mod  SaturateOnIntegerOverflow=on
  Maximum : dspstat3/Maximum  fcn=Index  reset=None  InputProcessing=Columns as channels (frame based)  indexBase=One  operateOver=Each column  Dimension=1  colComp=on  operation=maximum  roiEnable=off  roiType=Rectangles  roiPortion=Entire ROI  roiOutput=Individual statistics for each ROI  roiFlag=off  accumDataTypeStr=Inherit: Same as product output  accumLastDataTypeStr=Inherit: Same as product output  roundingMode=Floor  overflowMode=off
  Probe : Probe  ProbeSampleTime=off  ProbeComplexSignal=off
  Sum : Sum  Inputs=|-+  SaturateOnIntegerOverflow=on  InputSameDT=on  OutDataTypeStr=Inherit: Same as first input
  Sum1 : Sum  Inputs=|+-  SaturateOnIntegerOverflow=on  InputSameDT=on  OutDataTypeStr=Inherit: Same as first input
  Delay : Outport
  wires:
  Abs/1 -> Maximum/1
  Constant1/1 -> Sum1/2
  Sum1/1 -> Math Function/2
  Math Function/1 -> Delay/1
  Sum/1 -> Math Function/1
  Probe/1 -> Sum1/1, Sum/2
  Correlation/1 -> Abs/1
  Maximum/1 -> Sum/1
  Barker Reference/1 -> Correlation/1
  Data/1 -> Correlation/2, Probe/1

== system commqpskrx/Receiver/Data Decoding/Descrambling ==
  In : Inport
  Descrambler : commsequence2/Descrambler  M=2  poly=[1 1 1 0 1]  ini_sta=[0 0 0 0]
  Selector : Selector  IndexOptions=Index vector (dialog)  Indices=[qpsktxrx.BarkerLength*log2(qpsktxrx.M)+1:qpsktxrx.FrameSize*log2(qpsktxrx.M)]  OutputSizes=1
  Selector1 : Selector  IndexOptions=Index vector (dialog)  Indices=[1:qpsktxrx.MessageLength]  OutputSizes=1
  Out : Outport
  wires:
  Descrambler/1 -> Selector1/1
  Selector1/1 -> Out/1
  In/1 -> Selector/1
  Selector/1 -> Descrambler/1

== system commqpskrx/Receiver/Data Decoding/Phase Ambiguity Correction & Demodulation ==
  note: Phase Ambiguity Resolution
      | and Demodulation
  Phase : Inport
  Data : Inport  Port=2
  Complex Phase Shift : commutil2/Complex Phase Shift
  Gain : Gain  Gain=-1  OutDataTypeStr=Inherit: Same as input
  QPSK Demodulator Baseband : commdigbbndpm3/QPSK Demodulator Baseband  Ph=pi/4  Dec=Gray  OutType=Bit  DecType=Hard decision  VarSource=Dialog  Variance=1  outDtype1=Inherit via internal rule  outDtype2=Inherit via internal rule  derotateFactorWordLen=16
  Out : Outport
  wires:
  Phase/1 -> Gain/1
  Data/1 -> Complex Phase Shift/1
  Complex Phase Shift/1 -> QPSK Demodulator Baseband/1
  QPSK Demodulator Baseband/1 -> Out/1
  Gain/1 -> Complex Phase Shift/2

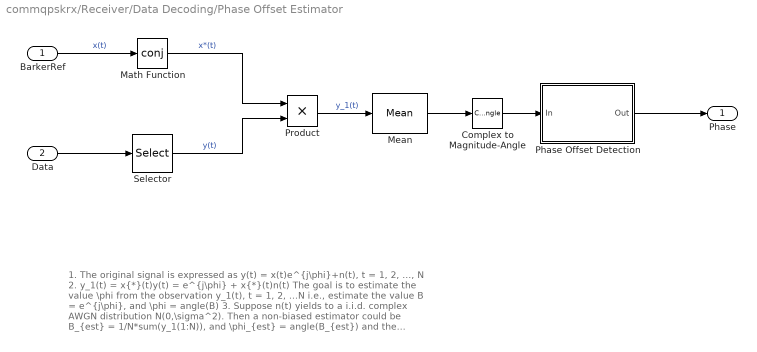
== system commqpskrx/Receiver/Data Decoding/Phase Offset Estimator ==
  note: 1. The original signal is expressed as y(t) = x(t)e^{j\phi}+n(t), t = 1, 2, ..., N
      | 2. y_1(t) = x{*}(t)y(t) = e^{j\phi} + x{*}(t)n(t)
      | The goal is to estimate the value \phi from the observation y_1(t), t = 1, 2, ...N
      | i.e., estimate the value B = e^{j\phi}, and \phi = angle(B)
      | 3. Suppose n(t) yields to a i.i.d. complex AWGN distribution N(0,\sigma^2).
      | Then a non-biased estimator could be
      | B_{est} = 1/N*sum(y_1(1:N)), and \phi_{est} = angle(B_{est})
      | and the variance of B_{est} is \sigma^2/N
  BarkerRef : Inport
  Data : Inport  Port=2
  Complex to Magnitude-Angle : ComplexToMagnitudeAngle  Output=Angle
  Math Function : Math  Operator=conj  SaturateOnIntegerOverflow=on
  Mean : dspstat3/Mean  run=off  reset_popup=None  InputProcessing=Columns as channels (frame based)  directionMode=Each column  dimension=1  treatSBRowAsCol=on  roiEnable=off  roiType=Rectangles  roiPortion=Entire ROI  roiOutput=Individual statistics for each ROI  roiFlag=off  outputDataTypeStr=Inherit: Same as accumulator  outputLastDataTypeStr=Inherit: Same as accumulator  outputMin=[]  outputMax=[]  roundingMode=Floor  overflowMode=off
  Phase Offset Detection : MATLAB Function  TreatAsAtomicUnit=on
  Product : Product  RndMeth=Zero
  Selector : Selector  IndexOptions=Index vector (dialog)  Indices=[1:qpsktxrx.BarkerLength]  OutputSizes=1
  Phase : Outport
  wires:
  Data/1 -> Selector/1
  BarkerRef/1 -> Math Function/1  "x(t)"
  Selector/1 -> Product/2  "y(t)"
  Math Function/1 -> Product/1  "x*(t)"
  Product/1 -> Mean/1  "y_1(t)"
  Mean/1 -> Complex to Magnitude-Angle/1
  Complex to Magnitude-Angle/1 -> Phase Offset Detection/1(In)
  Phase Offset Detection/1(Out) -> Phase/1

== system commqpskrx/Receiver/Fine Frequency Compensation/DDS ==
  note: The digital filter acts as a pure integrator
  In : Inport
  Digital Filter : dsparch4/Digital Filter  TypePopup=IIR (poles & zeros)  IIRFiltStruct=Direct form II transposed  AllPoleFiltStruct=Direct form  FIRFiltStruct=Direct form  CoeffSource=Specify via dialog  NumCoeffs=[0 1]  DenCoeffs=[1 -1]  BiQuadCoeffs=[1 0.3 0.4 1 0.1 0.2]  LatticeCoeffs=[0.2 0.4]  denIgnore=on  FiltPerSampPopup=One filter per frame  IC=0  ICnum=0  ICden=0  roundingMode=Floor  overflowMode=off  ScaleValues=1  scaleValueFracLength=14  stageInFracLength=15  stageOutFracLength=15  FilterSource=Specify via dialog  dfiltObjectName=dfilt.dffir([1 2 1])  InputProcessing=Columns as channels (frame based)
  Gain : Gain  Gain=-1*qpsktxrx.PhaseRecoveryGain
  Phase : Outport
  wires:
  Digital Filter/1 -> Gain/1
  In/1 -> Digital Filter/1
  Gain/1 -> Phase/1

== system commqpskrx/Receiver/Fine Frequency Compensation/Loop Filter ==
  note: Proportional-plus-Integrator Loop Filter,
      | Infinite DC Response to guarantee convergence
  e : Inport
  Digital Filter : dsparch4/Digital Filter  TypePopup=IIR (poles & zeros)  IIRFiltStruct=Direct form II transposed  AllPoleFiltStruct=Direct form  FIRFiltStruct=Direct form  CoeffSource=Specify via dialog  NumCoeffs=[1 0]  DenCoeffs=[1 -1]  BiQuadCoeffs=[1 0.3 0.4 1 0.1 0.2]  LatticeCoeffs=[0.2 0.4]  denIgnore=on  FiltPerSampPopup=One filter per frame  IC=0  ICnum=0  ICden=0  roundingMode=Floor  overflowMode=off  ScaleValues=1  scaleValueFracLength=14  stageInFracLength=15  stageOutFracLength=15  FilterSource=Specify via dialog  dfiltObjectName=dfilt.dffir([1 2 1])  InputProcessing=Columns as channels (frame based)
  K1 : Gain  Gain=K1
  K2 : Gain  Gain=K2
  Sum2 : Sum  SaturateOnIntegerOverflow=on  InputSameDT=on  OutDataTypeStr=Inherit: Same as first input
  v : Outport
  wires:
  K2/1 -> Digital Filter/1
  Digital Filter/1 -> Sum2/2
  Sum2/1 -> v/1
  e/1 -> K2/1, K1/1
  K1/1 -> Sum2/1

== system commqpskrx/Receiver/Timing Recovery/Enabled Wire ==
  In : Inport
  Enable : EnablePort
  Out : Outport
  wires:
  In/1 -> Out/1

== system commqpskrx/Receiver/Timing Recovery/Modified Buffer ==
  Data : Inport
  Clk : Inport  Port=2
  Frame Conversion : FrameConversion  OutFrame=Sample-based
  Logical Operator : Logic  AllPortsSameDT=off  OutDataTypeStr=boolean
  Modified Buffer : Subsystem
  DataOut : Outport
  DataValid : Outport  Port=2
  wires:
  Data/1 -> Modified Buffer/1(In)
  Modified Buffer/1(DataOut) -> Frame Conversion/1
  Modified Buffer/2(DataValid) -> Logical Operator/1
  Logical Operator/1 -> DataValid/1
  Frame Conversion/1 -> DataOut/1
  Clk/1 -> Modified Buffer/Enable, Logical Operator/2

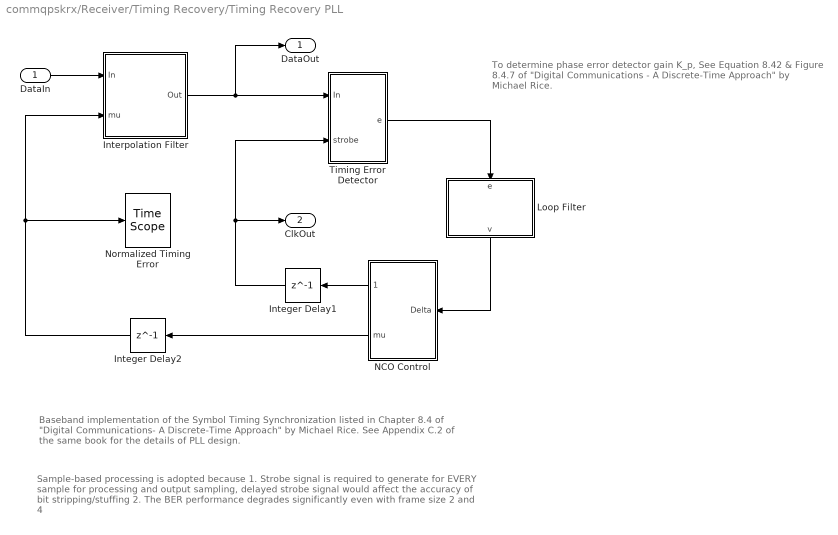
== system commqpskrx/Receiver/Timing Recovery/Timing Recovery PLL ==
  note: Sample-based processing is adopted because
      | 1. Strobe signal is required to generate for EVERY sample for processing and output
      | sampling, delayed strobe signal would affect the accuracy of bit stripping/stuffing
      | 2. The BER performance degrades significantly even with frame size 2 and 4
  note: Baseband implementation of the Symbol Timing Synchronization listed in Chapter 8.4
      | of "Digital Communications- A Discrete-Time Approach" by Michael Rice. See Appendix
      | C.2 of the same book for the details of PLL design.
  note: To determine phase error detector gain K_p, See Equation 8.42 &
      | Figure 8.4.7 of "Digital Communications - A Discrete-Time Approach"
      | by Michael Rice.
  DataIn : Inport
  Integer Delay1 : Delay  DelayLength=1  InputProcessing=Inherited
  Integer Delay2 : Delay  DelayLength=1  InputProcessing=Inherited
  Interpolation Filter : MATLAB Function  TreatAsAtomicUnit=on
  Loop Filter : Subsystem  mask{BnTs=0.01, zeta=1, Kp=qpsktxrx.TimingErrorDetectorGain, K0=qpsktxrx.TimingRecoveryGain, N=qpsktxrx.Upsampling/qpsktxrx.Downsampling}
      mask prompts: BnTs "Loop Bandwidth"; zeta "Loop Damping Factor"; Kp "Phase Detector Gain (Kp)"; K0 "DDS gain (K0)"; N "Number of Samples/symbol (N)"
      mask init:
      | % See C.57 to C.61 in Michael Rice's "Digital Communications 
      | % - A Discrete-Time Approach" for details
      | theta = BnTs/(zeta+0.25/zeta)/N;
      | d = 1 + 2*zeta*theta + theta*theta;
      | K1 = 4*zeta*theta/d;
      | K2 = 4*theta*theta/d;
      | K1 = K1/(Kp*K0);
      | K2 = K2/(Kp*K0);
      mask Display: disp('Loop Filter');
  NCO Control : MATLAB Function
  Normalized Timing Error : TimeScope  DefaultConfigurationName=spbscopes.TimeScopeBlockCfg
      settings: CopyFcn=scopeextensions.ScopeBlock.onCoreBlockCopy(gcbh);  DeleteFcn=scopeextensions.ScopeBlock.callback(gcbh, 'onBlockDelete');  PreSaveFcn=scopeextensions.ScopeBlock.callback(gcbh, 'onModelSave');  NameChangeFcn=scopeextensions.ScopeBlock.callback(gcbh, 'onBlockRename');  DestroyFcn=scopeextensions.ScopeBlock.onBlockDestroy(gcbh)  CloseFcn=scopeextensions.ScopeBlock.callback(gcbh, 'onBlockClose');  PreDeleteFcn=scopeextensions.ScopeBlock.callback(gcbh, 'onBlockPreDelete');
  Timing Error Detector : MATLAB Function  TreatAsAtomicUnit=on
  DataOut : Outport
  ClkOut : Outport  Port=2
  wires:
  DataIn/1 -> Interpolation Filter/1(In)
  NCO Control/2(mu) -> Integer Delay2/1
  Integer Delay1/1 -> ClkOut/1, Timing Error Detector/2(strobe)
  NCO Control/1(Underflow) -> Integer Delay1/1
  Interpolation Filter/1(Out) -> DataOut/1, Timing Error Detector/1(In)
  Loop Filter/1(v) -> NCO Control/1(Delta)
  Timing Error Detector/1(e) -> Loop Filter/1(e)
  Integer Delay2/1 -> Interpolation Filter/2(mu), Normalized Timing Error/1

== system commqpskrx/Transmitter/Bit Generation/Barker Code SS ==
  Constant Barker Code : Constant  Value=|  VectorParams1D=off  OutDataTypeStr=double
      | [+1 +1 +1 +1 +1 -1 -1 +1 +1 -1 +1 -1 +1
      | ].' > 0  % Bipolar to Unipolar Conversion
  Out : Outport
  wires:
  Constant Barker Code/1 -> Out/1

== system commqpskrx/Receiver/Timing Recovery/Modified Buffer/Modified Buffer ==
  In : Inport
  Enable : EnablePort
  Compare To Constant : simulink/Logic and Bit Operations/Compare To Constant  relop===  const=(bufSize-1)  OutDataTypeStr=boolean  ZeroCross=off
  Counter Limited : simulink/Sources/Counter Limited  uplimit=(bufSize-1)  tsamp=-1
  Delay Line : dspbuff3/Delay Line  siz=bufSize  ic=0  directfeed=on  enable_output=on  hold_output=off  TreatMby1Signals=One channel
  DataOut : Outport
  DataValid : Outport  Port=2
  wires:
  Compare To Constant/1 -> Delay Line/2, DataValid/1
  Delay Line/1 -> DataOut/1
  In/1 -> Delay Line/1
  Counter Limited/1 -> Compare To Constant/1

== system commqpskrx/Receiver/Timing Recovery/Timing Recovery PLL/Loop Filter ==
  note: Proportional-Plus-Integrator Loop Filter,
      | Infinite DC Response to guarantee convergence
  e : Inport
  Digital Filter : dsparch4/Digital Filter  TypePopup=IIR (poles & zeros)  IIRFiltStruct=Direct form II transposed  AllPoleFiltStruct=Direct form  FIRFiltStruct=Direct form  CoeffSource=Specify via dialog  NumCoeffs=[1 0]  DenCoeffs=[1 -1]  BiQuadCoeffs=[1 0.3 0.4 1 0.1 0.2]  LatticeCoeffs=[0.2 0.4]  denIgnore=on  FiltPerSampPopup=One filter per frame  IC=0  ICnum=0  ICden=0  roundingMode=Floor  overflowMode=off  ScaleValues=1  scaleValueFracLength=14  stageInFracLength=15  stageOutFracLength=15  FilterSource=Specify via dialog  dfiltObjectName=dfilt.dffir([1 2 1])  InputProcessing=Columns as channels (frame based)
  K1 : Gain  Gain=K1
  K2 : Gain  Gain=K2
  Sum2 : Sum  SaturateOnIntegerOverflow=on  InputSameDT=on  OutDataTypeStr=Inherit: Same as first input
  v : Outport
  wires:
  K2/1 -> Digital Filter/1
  Digital Filter/1 -> Sum2/2
  Sum2/1 -> v/1
  e/1 -> K2/1, K1/1
  K1/1 -> Sum2/1

== matlab function commqpskrx/Receiver/Timing Recovery/Calculate Number of Valid Samples ==
  data: Clk input; numValid output
function numValid = numValidCalc(Clk)
% Calculate the number of valid outputs in the current received frame. The
% typical value is 100 valid outputs in a 200-element frame. However, in
% bit stuffing case we have 101 valid outputs, and in bit stripping case we 
% have 99 valid outputs.
%
% Input:
%   Clk - Strobe signal
% Output:
%   NumValid - Number of valid outputs in the current received frame 
%#codegen
numValid = sum(Clk~=0);
